simulink model "Separtly_dc_motor_and_ac_dc_converter"  (R2022b)
settings: Solver=VariableStepAuto  StartTime=0.0  StopTime=0.8  MaxStep=0.0001  RelTol=1e-3
libraries: spsThyristorLib x4, spsVoltageMeasurementLib x2, spsControlledVoltageSourceLib x1, spsParallelRLCBranchLib x1, spsACVoltageSourceLib x1, sps_lib x1
settings Model: Creator=ahmed  LastModifiedBy=ahmed

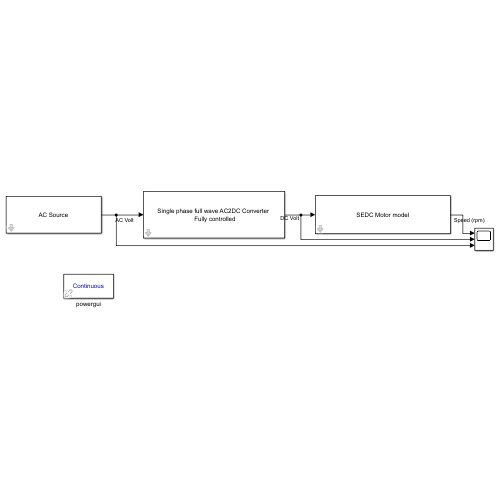
[thumbnail: Simulink's stored preview of the top-level diagram]
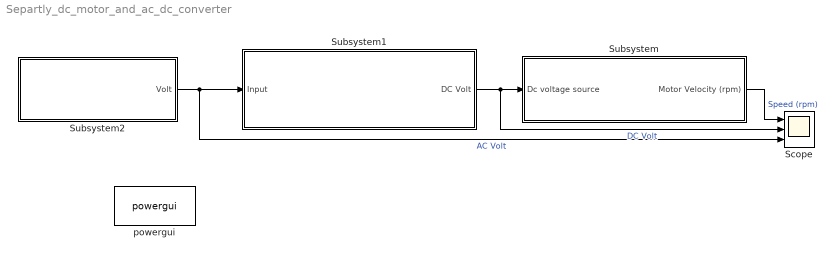
== system Separtly_dc_motor_and_ac_dc_converter ==
  Scope : Scope  NumInputPorts=3
  Subsystem : Subsystem  mask{TL=20, B=0.01, J=5, Ra=0.5, La=0.1, Kphi=1.6}
      mask prompts: TL "Torque Load (N.m)"; B "Friction Cooficient (N.m.s)"; J "Mechanical Inertia (Kg.m^2)"; Ra "Armature Resistence (Ohm)"; La "Armature Indectanc (H)"; Kphi "Back emf Constan (N.m/A)"
      mask DialogControl DescGroupVar Prompt: Separtly dc motor
      mask DialogControl DescTextVar Prompt: this block used to simulate Separtly dc motor
      mask Display: disp('SEDC Motor model');
  Subsystem1 : Subsystem
      mask DialogControl DescGroupVar Prompt: Converter
      mask DialogControl DescTextVar Prompt: This bock conver the volt from ac to dc volt
      mask Display: disp('Single phase full wave AC2DC Converter \n Fully controlled');
  Subsystem2 : Subsystem  mask{freq=50, pek=311}
      mask prompts: freq "Frequency (Hz)"; pek "Peak amplitude (V)"
      mask DialogControl DescGroupVar Prompt: The Ac  source
      mask Display: disp('AC Source');
  powergui : sps_lib/powergui  Priority=1  SimulationMode=Continuous  SampleTime=50e-6  frequency=60  Iterations=50  frequencyindice=50  Pbase=100e6  ErrMax=1e-4  UnitsV=kV  UnitsW=MW  buscounter=0  FunctionMessages=off  echomessages=off  EnableUseOfTLC=off  CurrentSourceSwitches=off  DisableSnubberDevices=off  DisableRonSwitches=off  DisableVfSwitches=off  DisplayEquations=off  AutomaticDiscreteSolvers=off  SolverType=Tustin/Backward Euler (TBE)  Interpol=off  ExternalGateDelay=off  methode=off  Ts=100  x0status=blocks  SPID=on  SwTol=0  HookPort=off  NonlinearTolerance=1e-4  nMaxIteration=100  ContinueOnMaxIteration=off  RestoreLinks=warning  ResistiveCurrentMeasurement=off  Frange=[0:2:500]  Ylog=off  Xlog=on  ShowGrid=off  save=off  variable=ZData  structure=0  ZoomFFT=off  StartTime=0.0  cycles=1  DisplayStyle=1  fundamental=60  FreqAxis=off  MaxFrequency=1000  frequencyindicesteady=1  RmsSteady=1  display=off
  wires:
  Subsystem/1(Motor Velocity (rpm)) -> Scope/1  "Speed (rpm)"
  Subsystem1/1(DC Volt) -> Scope/2, Subsystem/1(Dc voltage source)  "DC Volt"
  Subsystem2/1(Volt) -> Subsystem1/1(Input), Scope/3  "AC Volt"

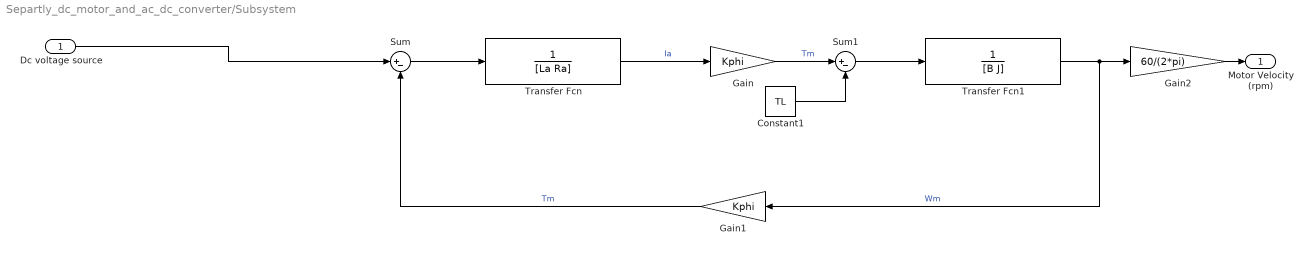
== system Separtly_dc_motor_and_ac_dc_converter/Subsystem ==
  Dc voltage source : Inport
  Constant1 : Constant  Value=TL
  Gain : Gain  Gain=Kphi
  Gain1 : Gain  Gain=Kphi
  Gain2 : Gain  Gain=60/(2*pi)
  Sum : Sum  Inputs=|+-
  Sum1 : Sum  Inputs=|+-
  Transfer Fcn : TransferFcn  Denominator=[La Ra]
  Transfer Fcn1 : TransferFcn  Denominator=[B J]
  Motor Velocity (rpm) : Outport
  wires:
  Gain2/1 -> Motor Velocity (rpm)/1
  Gain1/1 -> Sum/2  "Tm"
  Transfer Fcn1/1 -> Gain1/1, Gain2/1  "Wm"
  Sum/1 -> Transfer Fcn/1
  Gain/1 -> Sum1/1  "Tm"
  Constant1/1 -> Sum1/2
  Transfer Fcn/1 -> Gain/1  "Ia"
  Sum1/1 -> Transfer Fcn1/1
  Dc voltage source/1 -> Sum/1

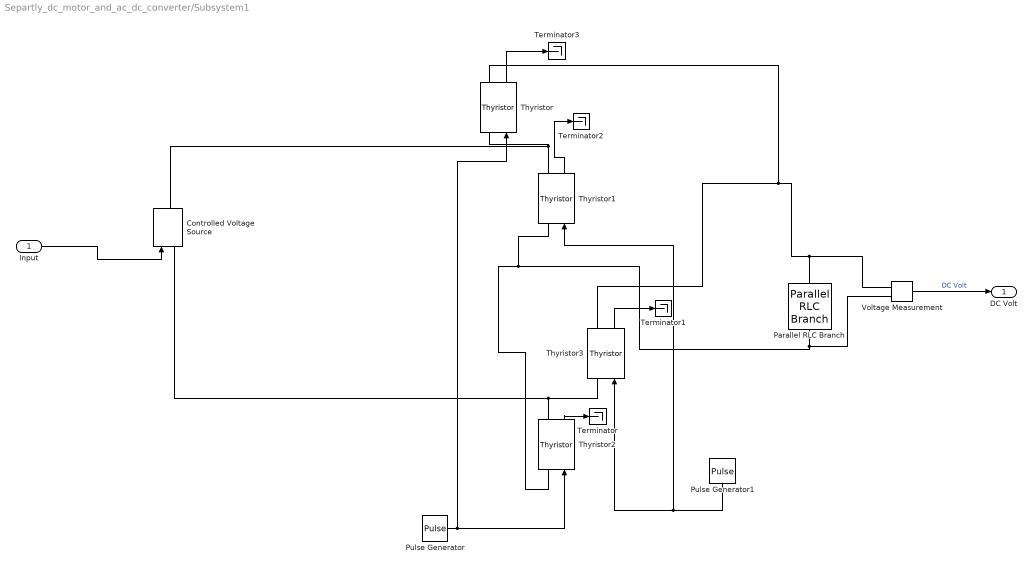
== system Separtly_dc_motor_and_ac_dc_converter/Subsystem1 ==
  Input : Inport
  Controlled Voltage Source : spsControlledVoltageSourceLib/Controlled Voltage Source  Initialize=on  Source_Type=AC  Amplitude=0  Phase=0  Frequency=0  Measurements=None
  Parallel RLC Branch : spsParallelRLCBranchLib/Parallel RLC Branch  LConnTagsString=a  RConnTagsString=__new0  BranchType=RC  Resistance=10000  Inductance=0.6  SetiL0=off  InitialCurrent=0  Capacitance=0.6  Setx0=off  InitialVoltage=0  Measurements=None
  Pulse Generator : DiscretePulseGenerator  PulseType=Time based  Period=0.02  PulseWidth=5  PhaseDelay=(0/360)*0.02
  Pulse Generator1 : DiscretePulseGenerator  PulseType=Time based  Period=0.02  PulseWidth=5  PhaseDelay=(180/360)*0.02
  Terminator{,1..3} (4 alike) : Terminator
  Thyristor{,1..3} (4 alike) : spsThyristorLib/Thyristor  Ron=0.001  Lon=0  Vf=0.8  IC=0  Rs=500  Cs=250e-9  Measurements=on
  Voltage Measurement : spsVoltageMeasurementLib/Voltage Measurement  PhasorSimulation=off  OutputType=Complex  PSBequivalent=0
  DC Volt : Outport
  wires:
  Voltage Measurement/1 -> DC Volt/1  "DC Volt"
  Pulse Generator/1 -> Thyristor/1, Thyristor2/1
  Thyristor/1 -> Terminator3/1
  Pulse Generator1/1 -> Thyristor3/1, Thyristor1/1
  Thyristor1/1 -> Terminator2/1
  Thyristor2/1 -> Terminator/1
  Thyristor3/1 -> Terminator1/1
  Input/1 -> Controlled Voltage Source/1
  connections:
  Parallel RLC Branch/RConn1 -- Voltage Measurement/LConn2 -- Thyristor2/LConn1 -- Thyristor1/LConn1
  Thyristor/RConn1 -- Thyristor3/RConn1 -- Voltage Measurement/LConn1 -- Parallel RLC Branch/LConn1
  Thyristor/LConn1 -- Controlled Voltage Source/RConn1 -- Thyristor1/RConn1
  Thyristor2/RConn1 -- Controlled Voltage Source/LConn1 -- Thyristor3/LConn1

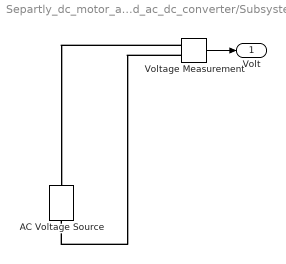
== system Separtly_dc_motor_and_ac_dc_converter/Subsystem2 ==
  AC Voltage Source : spsACVoltageSourceLib/AC Voltage Source  Amplitude=pek  Phase=0  Frequency=freq  SampleTime=0  Measurements=None  BusType=swing  Pref=10e3  Qref=0  Qmin=-inf  Qmax=+inf
  Voltage Measurement : spsVoltageMeasurementLib/Voltage Measurement  PhasorSimulation=off  OutputType=Complex  PSBequivalent=0
  Volt : Outport
  wires:
  Voltage Measurement/1 -> Volt/1
  connections:
  Voltage Measurement/LConn2 -- AC Voltage Source/LConn1
  Voltage Measurement/LConn1 -- AC Voltage Source/RConn1
